simulink model "complex_multiply_example"  (R2019b)
settings: Solver=FixedStepDiscrete  StartTime=0.0  StopTime=20  RelTol=1e-3
PostLoadFcn:
  | D1 = 1;
  | D2 = 1;
  | D3 = 1;
  | D4 = 1;
  | D5 = 1;
settings Model: DataTypeOverride=Off  Creator=cchung  LastModifiedBy=bhisma
settings DataIOCC: LimitDataPoints=on  SaveFormat=Array  SaveOutput=off  SaveTime=off  ReturnWorkspaceOutputs=off
settings OptimizationCC: BlockReduction=off  BooleanDataType=off  ConditionallyExecuteInputs=off  DefaultParameterBehavior=Inlined  LifeSpan=inf
settings DebuggingCC: AlgebraicLoopMsg=error  SaveWithParameterizedLinksMsg=none  UnderspecifiedInitializationDetection=Classic  MergeDetectMultiDrivingBlocksExec=none  SignalResolutionControl=TryResolveAllWithWarning  SingleTaskRateTransMsg=error  StrictBusMsg=ErrorOnBusTreatedAsVector  SFUnexpectedBacktrackingDiag=warning  SFNoUnconditionalDefaultTransitionDiag=warning  SFExecutionAtInitializationDiag=none  ArithmeticOperatorsInVariantConditions=warning
settings HardwareCC: ProdBitPerPointer=32  ProdBitPerSizeT=32  ProdBitPerPtrDiffT=32  ProdLargestAtomicFloat=None  ProdIntDivRoundTo=Undefined  ProdEndianess=Unspecified  ProdWordSize=32  ProdHWDeviceType=ASIC/FPGA->ASIC/FPGA  TargetUnknown=on  ProdEqTarget=off
settings ModelReferenceCC: PropagateSignalLabelsOutOfModel=off
settings SFSimCC: SimUseLocalCustomCode=off  CustomCodeUndefinedFunction=UseInterfaceOnly
settings RTWCC: RTWUseLocalCustomCode=off
settings CodeAppCC: StateflowObjectComments=on
settings GRTTargetCC: TargetLangStandard=C89/C90 (ANSI)  GeneratePreprocessorConditionals=Disable all
settings ConfigComp: CovMetricSettings=dw  CovHtmlReporting=on  CovSaveCumulativeToWorkspaceVar=on  CovSaveSingleToWorkspaceVar=on  CovExternalEMLEnable=off

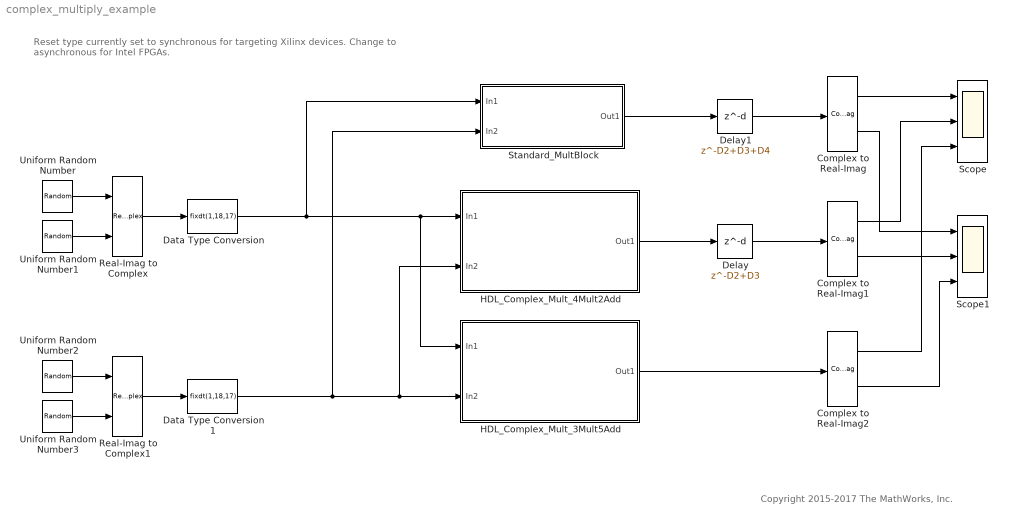
== system complex_multiply_example ==
  note: Copyright 2015-2017 The MathWorks, Inc.
  note: Reset type currently set to synchronous for targeting Xilinx devices.
      | Change to asynchronous for Intel FPGAs.
  Complex to Real-Imag : ComplexToRealImag
  Complex to Real-Imag1 : ComplexToRealImag
  Complex to Real-Imag2 : ComplexToRealImag
  Data Type Conversion : DataTypeConversion  OutDataTypeStr=fixdt(1,18,17)
  Data Type Conversion1 : DataTypeConversion  OutDataTypeStr=fixdt(1,18,17)
  Delay : Delay  DelayLength=D2+D3
  Delay1 : Delay  DelayLength=D2+D3+D4
  HDL_Complex_Mult_3Mult5Add : Subsystem
  HDL_Complex_Mult_4Mult2Add : Subsystem
  Real-Imag to Complex : RealImagToComplex
  Real-Imag to Complex1 : RealImagToComplex
  Scope : Scope  NumInputPorts=3
  Scope1 : Scope  NumInputPorts=3
  Standard_MultBlock : Subsystem
  Uniform Random Number : UniformRandomNumber  Minimum=0  SampleTime=1
  Uniform Random Number1 : UniformRandomNumber  Minimum=0  Seed=1  SampleTime=1
  Uniform Random Number2 : UniformRandomNumber  Minimum=0  Seed=2  SampleTime=1
  Uniform Random Number3 : UniformRandomNumber  Minimum=0  Seed=3  SampleTime=1
  wires:
  HDL_Complex_Mult_4Mult2Add/1(Out1) -> Delay/1
  Data Type Conversion/1 -> Standard_MultBlock/1(In1), HDL_Complex_Mult_3Mult5Add/1(In1), HDL_Complex_Mult_4Mult2Add/1(In1)
  Data Type Conversion1/1 -> Standard_MultBlock/2(In2), HDL_Complex_Mult_4Mult2Add/2(In2), HDL_Complex_Mult_3Mult5Add/2(In2)
  Standard_MultBlock/1(Out1) -> Delay1/1
  HDL_Complex_Mult_3Mult5Add/1(Out1) -> Complex to Real-Imag2/1
  Real-Imag to Complex/1 -> Data Type Conversion/1
  Uniform Random Number/1 -> Real-Imag to Complex/1
  Uniform Random Number1/1 -> Real-Imag to Complex/2
  Real-Imag to Complex1/1 -> Data Type Conversion1/1
  Uniform Random Number2/1 -> Real-Imag to Complex1/1
  Uniform Random Number3/1 -> Real-Imag to Complex1/2
  Complex to Real-Imag/1 -> Scope/1
  Complex to Real-Imag1/1 -> Scope/2
  Complex to Real-Imag2/1 -> Scope/3
  Complex to Real-Imag2/2 -> Scope1/3
  Complex to Real-Imag1/2 -> Scope1/2
  Complex to Real-Imag/2 -> Scope1/1
  Delay/1 -> Complex to Real-Imag1/1
  Delay1/1 -> Complex to Real-Imag/1

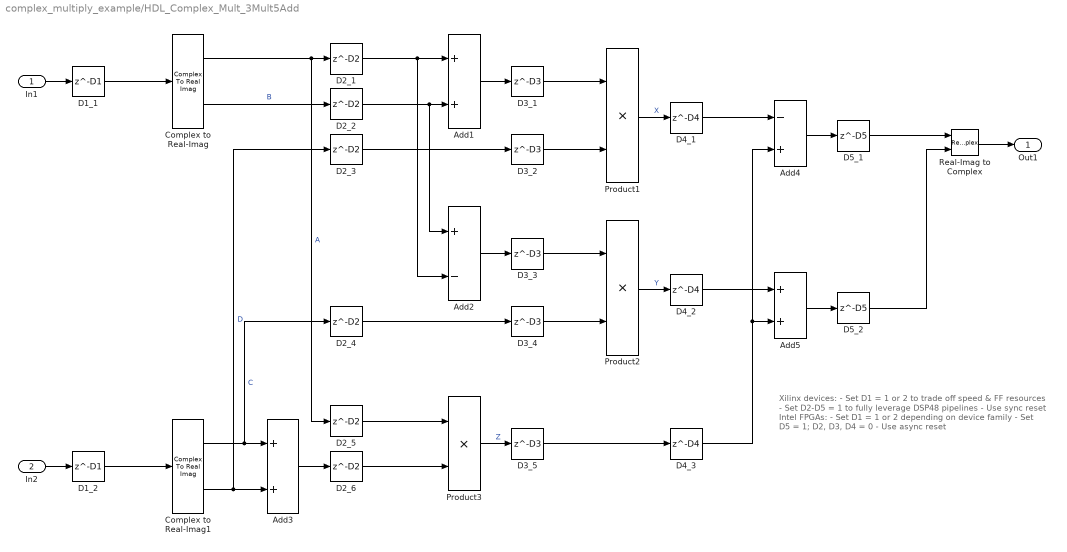
== system complex_multiply_example/HDL_Complex_Mult_3Mult5Add ==
  note: Xilinx devices:
      | - Set D1 = 1 or 2 to trade off speed & FF resources
      | - Set D2-D5 = 1 to fully leverage DSP48 pipelines
      | - Use sync reset
      |
      | Intel FPGAs:
      | - Set D1 = 1 or 2 depending on device family
      | - Set D5 = 1; D2, D3, D4 = 0
      | - Use async reset
  In1 : Inport
  In2 : Inport  Port=2
  Add1 : Sum
  Add2 : Sum  Inputs=+-
  Add3 : Sum
  Add4 : Sum  Inputs=-+
  Add5 : Sum
  Complex to Real-Imag : ComplexToRealImag
  Complex to Real-Imag1 : ComplexToRealImag
  D1_1 : Delay  DelayLength=D1
  D1_2 : Delay  DelayLength=D1
  D2_{1..6} (6 alike) : Delay  DelayLength=D2
  D3_{1..5} (5 alike) : Delay  DelayLength=D3
  D4_1 : Delay  DelayLength=D4
  D4_2 : Delay  DelayLength=D4
  D4_3 : Delay  DelayLength=D4
  D5_1 : Delay  DelayLength=D5
  D5_2 : Delay  DelayLength=D5
  Product1 : Product
  Product2 : Product
  Product3 : Product
  Real-Imag to Complex : RealImagToComplex
  Out1 : Outport
  wires:
  Real-Imag to Complex/1 -> Out1/1
  In2/1 -> D1_2/1
  Complex to Real-Imag1/1 -> Add3/1, D2_4/1  "C"
  Complex to Real-Imag1/2 -> Add3/2, D2_3/1  "D"
  Product1/1 -> D4_1/1  "X"
  Product2/1 -> D4_2/1  "Y"
  Product3/1 -> D3_5/1  "Z"
  Add4/1 -> D5_1/1
  Add5/1 -> D5_2/1
  D5_1/1 -> Real-Imag to Complex/1
  D5_2/1 -> Real-Imag to Complex/2
  D4_1/1 -> Add4/1
  D4_2/1 -> Add5/1
  D3_5/1 -> D4_3/1
  Add1/1 -> D3_1/1
  Add3/1 -> D2_6/1
  Add2/1 -> D3_3/1
  Complex to Real-Imag/1 -> D2_5/1, D2_1/1  "A"
  Complex to Real-Imag/2 -> D2_2/1  "B"
  D3_1/1 -> Product1/1
  D2_6/1 -> Product3/2
  D3_3/1 -> Product2/1
  D4_3/1 -> Add4/2, Add5/2
  D3_4/1 -> Product2/2
  D3_2/1 -> Product1/2
  D2_4/1 -> D3_4/1
  D2_3/1 -> D3_2/1
  D2_5/1 -> Product3/1
  D2_2/1 -> Add1/2, Add2/1
  D2_1/1 -> Add2/2, Add1/1
  In1/1 -> D1_1/1
  D1_1/1 -> Complex to Real-Imag/1
  D1_2/1 -> Complex to Real-Imag1/1

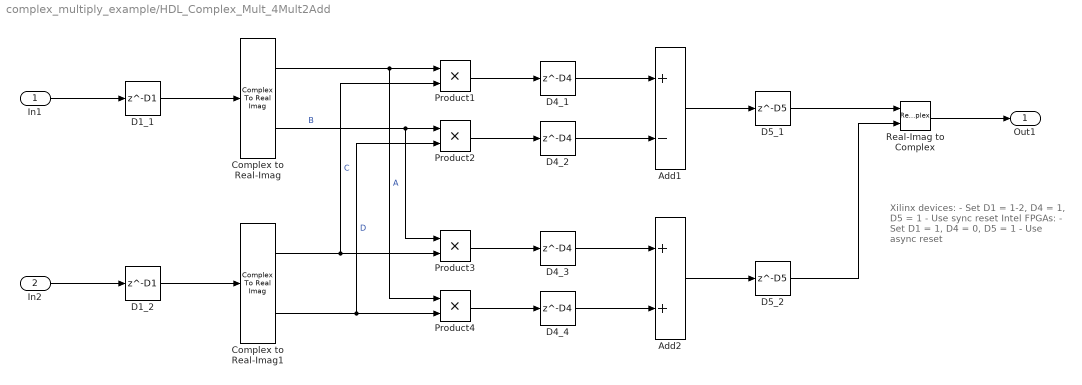
== system complex_multiply_example/HDL_Complex_Mult_4Mult2Add ==
  note: Xilinx devices:
      | - Set D1 = 1-2, D4 = 1, D5 = 1
      | - Use sync reset
      |
      | Intel FPGAs:
      | - Set D1 = 1, D4 = 0, D5 = 1
      | - Use async reset
  In1 : Inport
  In2 : Inport  Port=2
  Add1 : Sum  Inputs=+-
  Add2 : Sum
  Complex to Real-Imag : ComplexToRealImag
  Complex to Real-Imag1 : ComplexToRealImag
  D1_1 : Delay  DelayLength=D1
  D1_2 : Delay  DelayLength=D1
  D4_{1..4} (4 alike) : Delay  DelayLength=D4
  D5_1 : Delay  DelayLength=D5
  D5_2 : Delay  DelayLength=D5
  Product{1..4} (4 alike) : Product
  Real-Imag to Complex : RealImagToComplex
  Out1 : Outport
  wires:
  In2/1 -> D1_2/1
  In1/1 -> D1_1/1
  Real-Imag to Complex/1 -> Out1/1
  D1_1/1 -> Complex to Real-Imag/1
  D1_2/1 -> Complex to Real-Imag1/1
  Complex to Real-Imag/1 -> Product4/1, Product1/1  "A"
  Complex to Real-Imag1/1 -> Product3/2, Product1/2  "C"
  Complex to Real-Imag/2 -> Product3/1, Product2/1  "B"
  Complex to Real-Imag1/2 -> Product4/2, Product2/2  "D"
  Product1/1 -> D4_1/1
  Product3/1 -> D4_3/1
  Add1/1 -> D5_1/1
  Add2/1 -> D5_2/1
  D5_1/1 -> Real-Imag to Complex/1
  D5_2/1 -> Real-Imag to Complex/2
  D4_1/1 -> Add1/1
  Product2/1 -> D4_2/1
  D4_3/1 -> Add2/1
  Product4/1 -> D4_4/1
  D4_2/1 -> Add1/2
  D4_4/1 -> Add2/2

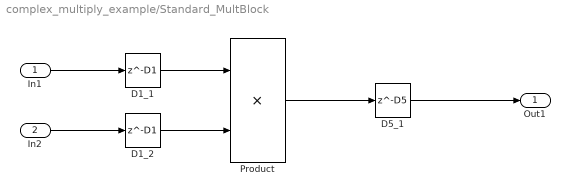
== system complex_multiply_example/Standard_MultBlock ==
  In1 : Inport
  In2 : Inport  Port=2
  D1_1 : Delay  DelayLength=D1
  D1_2 : Delay  DelayLength=D1
  D5_1 : Delay  DelayLength=D5
  Product : Product  OutDataTypeStr=fixdt(1,37,34)
  Out1 : Outport
  wires:
  Product/1 -> D5_1/1
  D5_1/1 -> Out1/1
  In1/1 -> D1_1/1
  In2/1 -> D1_2/1
  D1_1/1 -> Product/1
  D1_2/1 -> Product/2
